simulink model "LgV2"  (Simulink 7.3)
settings: Solver=ode5  StartTime=0.0  StopTime=inf  FixedStep=0.1  RelTol=1e-3
undefined symbols (not defined in the file): eta1_0_real, v1_0_real, velocitySatValues1
libraries: simulink x35, dspmtrx3 x21, simulink_extras x13, dspindex x5, marine_gnc x4, dspinverses x2
(part 2 of 5)

== system LgV2/Control Systems/LgV design 2/Auxilary functions g_q ==
  f_q : Inport
  psi_los^q : Inport  Port=2
  f_q^q : Inport  Port=3
  psi_los^q^2 : Inport  Port=4
  f_q^s : Inport  Port=5
  psi_los^qs : Inport  Port=6
  f_q^t : Inport  Port=7
  g_q eq : Subsystem
  g_q^q eq : Subsystem
  g_q^s eq : Subsystem
  g_q^t eq : Subsystem
  g_q : Outport
  g_q^t : Outport  Port=2
  g_q^q : Outport  Port=3
  g_q^s : Outport  Port=4
  wires:
  g_q eq/1(g_q) -> g_q/1
  psi_los^q/1 -> g_q eq/2(psi_los^q), g_q^q eq/2(psi_los^q), g_q^s eq/2(psi_los^q), g_q^t eq/1(psi_los^q)
  f_q/1 -> g_q eq/1(f_q), g_q^q eq/1(f_q), g_q^s eq/1(f_q)
  f_q^q/1 -> g_q^q eq/3(f_q^q)
  psi_los^q^2/1 -> g_q^q eq/4(psi_los^q^2)
  g_q^q eq/1(g_q^q) -> g_q^q/1
  g_q^s eq/1(g_q^s) -> g_q^s/1
  f_q^s/1 -> g_q^s eq/3(f_q^s)
  psi_los^qs/1 -> g_q^s eq/4(psi_los^qs)
  g_q^t eq/1(g_q^t) -> g_q^t/1
  f_q^t/1 -> g_q^t eq/2(f_q^t)

== system LgV2/Control Systems/LgV design 2/Auxiliary function g_s ==
  psi_los^sq : Inport
  f_s : Inport  Port=2
  psi_los^s : Inport  Port=3
  f_s^q : Inport  Port=4
  f_s^s : Inport  Port=5
  psi_los^s^2 : Inport  Port=6
  f_s^t : Inport  Port=7
  g_s eq : Subsystem
  g_s^q eq : Subsystem
  g_s^s eq : Subsystem
  g_s^t eq : Subsystem
  g_s^q : Outport
  g_s^s : Outport  Port=2
  g_s^t : Outport  Port=3
  g_s : Outport  Port=4
  wires:
  f_s/1 -> g_s eq/1(f_s), g_s^q eq/1(f_s), g_s^s eq/1(f_s)
  psi_los^s/1 -> g_s eq/2(psi_los^s), g_s^q eq/2(psi_los^s), g_s^s eq/2(psi_los^s), g_s^t eq/1(psi_los^s)
  g_s eq/1(g_s) -> g_s/1
  f_s^q/1 -> g_s^q eq/3(f_s^q)
  psi_los^sq/1 -> g_s^q eq/4(psi_los^sq)
  g_s^q eq/1(g_s^q) -> g_s^q/1
  g_s^s eq/1(g_s^s) -> g_s^s/1
  f_s^s/1 -> g_s^s eq/3(f_s^s)
  psi_los^s^2/1 -> g_s^s eq/4(psi_los^s^2)
  g_s^t eq/1(g_a^t) -> g_s^t/1
  f_s^t/1 -> g_s^t eq/2(f_s^t)

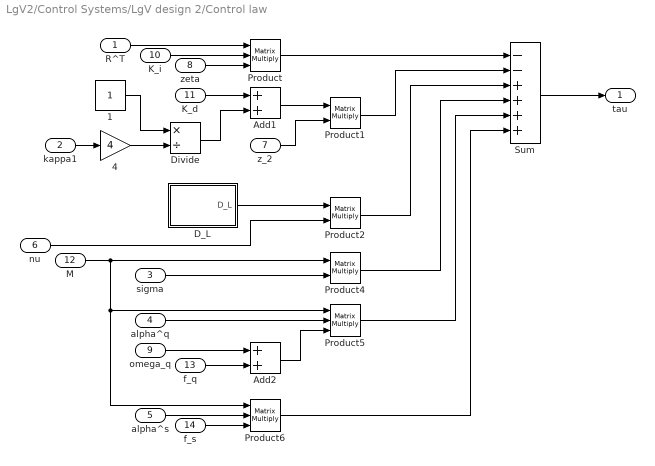
== system LgV2/Control Systems/LgV design 2/Control law ==
  R^T : Inport
  kappa1 : Inport  Port=2
  sigma : Inport  Port=3
  alpha^q : Inport  Port=4
  alpha^s : Inport  Port=5
  nu : Inport  Port=6
  z_2 : Inport  Port=7
  zeta : Inport  Port=8
  omega_q : Inport  Port=9
  K_i : Inport  Port=10
  K_d : Inport  Port=11
  M : Inport  Port=12
  f_q : Inport  Port=13
  f_s : Inport  Port=14
  1 : Constant  OutDataType=fixdt(1, 16)  OutScaling=2^0
  4 : Gain  Gain=4  ParameterDataType=fixdt(1, 16)  ParameterScaling=2^0  OutDataType=fixdt(1, 16)  OutScaling=2^0
  Add1 : Sum  OutDataType=fixdt(1, 16)  OutScaling=2^-10
  Add2 : Sum  OutDataType=fixdt(1, 16)  OutScaling=2^-10
  D_L : Subsystem
  Divide : Product  Inputs=*/  OutDataType=fixdt(1, 16)  OutScaling=2^-10
  Product : Product  Inputs=3  Multiplication=Matrix(*)  OutDataType=fixdt(1, 16)  OutScaling=2^0  RndMeth=Zero
  Product1 : Product  Multiplication=Matrix(*)  OutDataType=fixdt(1, 16)  OutScaling=2^0  RndMeth=Zero
  Product2 : Product  Multiplication=Matrix(*)  OutDataType=fixdt(1, 16)  OutScaling=2^0  RndMeth=Zero
  Product4 : Product  Multiplication=Matrix(*)  OutDataType=fixdt(1, 16)  OutScaling=2^0  RndMeth=Zero
  Product5 : Product  Inputs=3  Multiplication=Matrix(*)  OutDataType=fixdt(1, 16)  OutScaling=2^0  RndMeth=Zero
  Product6 : Product  Inputs=3  Multiplication=Matrix(*)  OutDataType=fixdt(1, 16)  OutScaling=2^0  RndMeth=Zero
  Sum : Sum  Inputs=--++++  OutDataType=fixdt(1, 16)  OutScaling=2^-10
  tau : Outport
  wires:
  Sum/1 -> tau/1
  R^T/1 -> Product/1
  K_i/1 -> Product/2
  zeta/1 -> Product/3
  K_d/1 -> Add1/1
  Divide/1 -> Add1/2
  1/1 -> Divide/1
  kappa1/1 -> 4/1
  4/1 -> Divide/2
  Add1/1 -> Product1/1
  z_2/1 -> Product1/2
  Product1/1 -> Sum/2
  nu/1 -> Product2/2
  D_L/1(D_L) -> Product2/1
  Product2/1 -> Sum/3
  M/1 -> Product4/1, Product5/1, Product6/1
  sigma/1 -> Product4/2
  Product4/1 -> Sum/4
  alpha^q/1 -> Product5/2
  Product5/1 -> Sum/5
  alpha^s/1 -> Product6/2
  f_s/1 -> Product6/3
  Product6/1 -> Sum/6
  omega_q/1 -> Add2/1
  f_q/1 -> Add2/2
  Add2/1 -> Product5/3
  Product/1 -> Sum/1

== system LgV2/Control Systems/LgV design 2/Gamma_q ==
  11 : Inport
  22 : Inport  Port=2
  12 : Constant  Value=0
  21 : Constant  Value=0
  2x2 : Reshape  OutputDimensionality=Customize  OutputDimensions=[2,2]
  Mux : Mux
  Gamma_q : Outport
  wires:
  2x2/1 -> Gamma_q/1
  Mux/1 -> 2x2/1
  11/1 -> Mux/1
  21/1 -> Mux/2
  12/1 -> Mux/3
  22/1 -> Mux/4

== system LgV2/Control Systems/LgV design 2/Integral action state ==
  z_2 : Inport
  R : Inport  Port=2
  Integrator : Integrator  InitialCondition=[0 0 0]'
  Product : Product  Multiplication=Matrix(*)  OutDataType=fixdt(1, 16)  OutScaling=2^0  RndMeth=Zero
  zeta : Outport
  wires:
  R/1 -> Product/1
  z_2/1 -> Product/2
  Integrator/1 -> zeta/1
  Product/1 -> Integrator/1

== system LgV2/Control Systems/LgV design 2/K_d ==
  11 : Inport
  22 : Inport  Port=2
  33 : Inport  Port=3
  {12..13,21,23,31..32} (6 alike) : Constant  Value=0
  3x3 : Reshape  OutputDimensionality=Customize  OutputDimensions=[3,3]
  Mux : Mux  Inputs=9
  K_d : Outport
  wires:
  3x3/1 -> K_d/1
  Mux/1 -> 3x3/1
  11/1 -> Mux/1
  21/1 -> Mux/2
  31/1 -> Mux/3
  12/1 -> Mux/4
  22/1 -> Mux/5
  32/1 -> Mux/6
  13/1 -> Mux/7
  23/1 -> Mux/8
  33/1 -> Mux/9

== system LgV2/Control Systems/LgV design 2/K_i ==
  11 : Inport
  22 : Inport  Port=2
  33 : Inport  Port=3
  {12..13,21,23,31..32} (6 alike) : Constant  Value=0
  3x3 : Reshape  OutputDimensionality=Customize  OutputDimensions=[3,3]
  Mux : Mux  Inputs=9
  K_i : Outport
  wires:
  3x3/1 -> K_i/1
  Mux/1 -> 3x3/1
  11/1 -> Mux/1
  21/1 -> Mux/2
  31/1 -> Mux/3
  12/1 -> Mux/4
  22/1 -> Mux/5
  32/1 -> Mux/6
  13/1 -> Mux/7
  23/1 -> Mux/8
  33/1 -> Mux/9

== system LgV2/Control Systems/LgV design 2/K_p ==
  11 : Inport
  22 : Inport  Port=2
  33 : Inport  Port=3
  {12..13,21,23,31..32} (6 alike) : Constant  Value=0
  Mux : Mux  Inputs=9
  R(psi) : Reshape  OutputDimensionality=Customize  OutputDimensions=[3,3]
  K_p : Outport
  wires:
  R(psi)/1 -> K_p/1
  Mux/1 -> R(psi)/1
  11/1 -> Mux/1
  21/1 -> Mux/2
  31/1 -> Mux/3
  12/1 -> Mux/4
  22/1 -> Mux/5
  32/1 -> Mux/6
  13/1 -> Mux/7
  23/1 -> Mux/8
  33/1 -> Mux/9

== system LgV2/Control Systems/LgV design 2/M ==
  3x3 : Reshape  OutputDimensionality=Customize  OutputDimensions=[3,3]
  I_z : Constant  Value=1.760
  M_{11,22..23,32..33} (5 alike) : Sum  Inputs=+-
  M_{12..13,21,31} (4 alike) : Constant  Value=0
  Mux : Mux  Inputs=9
  N_rdot : Constant  Value=-1.0
  N_vdot : Constant  Value=-0.0
  X_udot : Constant  Value=-2.0
  Y_rdot : Constant  Value=0.0
  Y_vdot : Constant  Value=-10.0
  m : Constant  Value=17.6
  m x_g : Product  RndMeth=Zero
  x_g : Constant  Value=0.03
  M : Outport
  wires:
  3x3/1 -> M/1
  Mux/1 -> 3x3/1
  M_33/1 -> Mux/9
  M_23/1 -> Mux/8
  M_13/1 -> Mux/7
  M_32/1 -> Mux/6
  M_22/1 -> Mux/5
  M_12/1 -> Mux/4
  M_31/1 -> Mux/3
  M_21/1 -> Mux/2
  M_11/1 -> Mux/1
  N_rdot/1 -> M_33/2
  I_z/1 -> M_33/1
  Y_rdot/1 -> M_23/2
  N_vdot/1 -> M_32/2
  m x_g/1 -> M_23/1, M_32/1
  x_g/1 -> m x_g/2
  Y_vdot/1 -> M_22/2
  X_udot/1 -> M_11/2
  m/1 -> m x_g/1, M_22/1, M_11/1

== system LgV2/Control Systems/LgV design 2/R(psi) ==
  psi : Inport
  -1 : Gain  Gain=-1  ParameterDataType=fixdt(1, 16)  ParameterScaling=2^0  OutDataType=fixdt(1, 16)  OutScaling=2^0
  Mux : Mux  Inputs=9
  R(psi) : Reshape  OutputDimensionality=Customize  OutputDimensions=[3,3]
  R11 : Trigonometry  Operator=cos
  R12 : Trigonometry
  R{13,23,31..32} (4 alike) : Constant  Value=0
  R21 : Trigonometry
  R22 : Trigonometry  Operator=cos
  R33 : Constant
  R : Outport
  wires:
  R(psi)/1 -> R/1
  Mux/1 -> R(psi)/1
  psi/1 -> R11/1, R21/1, R12/1, R22/1
  R11/1 -> Mux/1
  R21/1 -> Mux/2
  R31/1 -> Mux/3
  R12/1 -> -1/1
  R22/1 -> Mux/5
  R32/1 -> Mux/6
  R13/1 -> Mux/7
  R33/1 -> Mux/9
  R23/1 -> Mux/8
  -1/1 -> Mux/4

== system LgV2/Control Systems/LgV design 2/S(r) ==
  r : Inport
  Mux : Mux  Inputs=9
  R31 : Constant  Value=0
  S(r) : Reshape  OutputDimensionality=Customize  OutputDimensions=[3,3]
  S{11,13,22..23,32} (5 alike) : Constant  Value=0
  S12 : Gain  ParameterDataType=fixdt(1, 16)  ParameterScaling=2^0  OutDataType=fixdt(1, 16)  OutScaling=2^0
  S33 : Constant
  S : Outport
  wires:
  S(r)/1 -> S/1
  Mux/1 -> S(r)/1
  R31/1 -> Mux/3
  S12/1 -> Mux/4
  S22/1 -> Mux/5
  S32/1 -> Mux/6
  S13/1 -> Mux/7
  S33/1 -> Mux/9
  S23/1 -> Mux/8
  r/1 -> Mux/2, S12/1
  S11/1 -> Mux/1

== system LgV2/Control Systems/LgV design 2/Thruster allocation ==
  tau : Inport
  f_act to u_act : Subsystem
  tau to f_act : Subsystem
  u_act : Outport
  wires:
  tau/1 -> tau to f_act/1(tau)
  tau to f_act/1(f_act) -> f_act to u_act/1(f_act)
  f_act to u_act/1(u_act) -> u_act/1

== system LgV2/Control Systems/LgV design 2/Update laws ==
  V_1^q : Inport
  Gamma_q : Inport  Port=2
  lambda : Inport  Port=3
  f_q : Inport  Port=4
  f_s : Inport  Port=5
  Add : Sum  OutDataType=fixdt(1, 16)  OutScaling=2^-10
  Add1 : Sum  OutDataType=fixdt(1, 16)  OutScaling=2^-10
  Gain : Gain  Gain=-1  ParameterDataType=fixdt(1, 16)  ParameterScaling=2^0  OutDataType=fixdt(1, 16)  OutScaling=2^0
  Integrator : Integrator  ExternalReset=level  InitialConditionSource=external
  Integrator1 : Integrator  ExternalReset=level  InitialConditionSource=external  InitialCondition=250
  Integrator2 : Integrator  ExternalReset=level
  Product : Product  Multiplication=Matrix(*)  OutDataType=fixdt(1, 16)  OutScaling=2^0  RndMeth=Zero
  Product1 : Product  OutDataType=fixdt(1, 16)  OutScaling=2^0  RndMeth=Zero
  Reset omega_q : Constant  Value=0
  Reset q : Constant  Value=0
  Reset s : Constant  Value=0
  Transpose : dspmtrx3/Transpose  SystemSampleTime=-1  Hermitian=off  overflowFlag=off
  q_0 : Subsystem
  s_0 : Constant  Value=0
  omega_q : Outport
  q : Outport  Port=2  PortDimensions=2
  s : Outport  Port=3  PortDimensions=1
  wires:
  f_q/1 -> Add/2
  Add/1 -> Integrator/1
  Product/1 -> Add1/2
  V_1^q/1 -> Transpose/1
  Gamma_q/1 -> Product/1
  lambda/1 -> Product1/1
  Add1/1 -> Product1/2
  Product1/1 -> Gain/1
  Gain/1 -> Integrator2/1
  f_s/1 -> Integrator1/1
  Transpose/1 -> Product/2
  Integrator/1 -> q/1
  Integrator1/1 -> s/1
  Integrator2/1 -> omega_q/1, Add/1, Add1/1
  Reset s/1 -> Integrator1/2
  s_0/1 -> Integrator1/3
  Reset q/1 -> Integrator/2
  q_0/1(q_0) -> Integrator/3
  Reset omega_q/1 -> Integrator2/2

== system LgV2/Control Systems/LgV design 2/V_1^q ==
  chi^q : Inport
  z_1 : Inport  Port=2
  R^T : Inport  Port=3
  Gain : Gain  Gain=-1  ParameterDataType=fixdt(1, 16)  ParameterScaling=2^0  OutDataType=fixdt(1, 16)  OutScaling=2^0
  Product : Product  Inputs=3  Multiplication=Matrix(*)  OutDataType=fixdt(1, 16)  OutScaling=2^0  RndMeth=Zero
  Transpose : dspmtrx3/Transpose  SystemSampleTime=-1  Hermitian=off  overflowFlag=off
  V_1^q : Outport
  wires:
  Product/1 -> Gain/1
  R^T/1 -> Product/2
  z_1/1 -> Transpose/1
  Transpose/1 -> Product/1
  chi^q/1 -> Product/3
  Gain/1 -> V_1^q/1

== system LgV2/Control Systems/LgV design 2/Virtual control ==
  g_q : Inport
  g_s : Inport  Port=2
  K_p : Inport  Port=3
  kappa_1 : Inport  Port=4
  R^T : Inport  Port=5
  z_1 : Inport  Port=6
  Add : Sum  OutDataType=fixdt(1, 16)  OutScaling=2^-10
  I : dspmtrx3/Constant Diagonal Matrix  SystemSampleTime=-1  q=[1 1 1 ]  frame=off  dataType=Inherit from 'Constant(s) along diagonal'  isSigned=on  wordLen=16  udDataType=sfix(16)  fracBitsMode=Best precision  numFracBits=15
  Product : Product  OutDataType=fixdt(1, 16)  OutScaling=2^0  RndMeth=Zero
  Product1 : Product  Multiplication=Matrix(*)  OutDataType=fixdt(1, 16)  OutScaling=2^0  RndMeth=Zero
  Product2 : Product  Multiplication=Matrix(*)  OutDataType=fixdt(1, 16)  OutScaling=2^0  RndMeth=Zero
  Subtract : Sum  Inputs=+-  OutDataType=fixdt(1, 16)  OutScaling=2^-10
  Sum : Sum  Inputs=-+  OutDataType=fixdt(1, 16)  OutScaling=2^-10
  alpha : Outport
  wires:
  Sum/1 -> alpha/1
  K_p/1 -> Subtract/1
  kappa_1/1 -> Product/1
  I/1 -> Product/2
  Product/1 -> Subtract/2
  Subtract/1 -> Product1/1
  z_1/1 -> Product1/2
  Product1/1 -> Sum/1
  R^T/1 -> Product2/1
  g_q/1 -> Add/1
  g_s/1 -> Add/2
  Add/1 -> Product2/2
  Product2/1 -> Sum/2

== system LgV2/Control Systems/LgV design 2/alpha^q ==
  kappa1 : Inport
  R^T : Inport  Port=2
  K_p : Inport  Port=3
  g_q^q : Inport  Port=4
  g_s^q : Inport  Port=5
  chi^q : Inport  Port=6
  Add : Sum  OutDataType=fixdt(1, 16)  OutScaling=2^-10
  Add2 : Sum  OutDataType=fixdt(1, 16)  OutScaling=2^-10
  Add3 : Sum  OutDataType=fixdt(1, 16)  OutScaling=2^-10
  I : dspmtrx3/Constant Diagonal Matrix  SystemSampleTime=-1  q=[1 1 1 ]  frame=off  dataType=Inherit from 'Constant(s) along diagonal'  isSigned=on  wordLen=16  udDataType=sfix(16)  fracBitsMode=Best precision  numFracBits=15
  Product1 : Product  OutDataType=fixdt(1, 16)  OutScaling=2^0  RndMeth=Zero
  Product3 : Product  Inputs=3  Multiplication=Matrix(*)  OutDataType=fixdt(1, 16)  OutScaling=2^0  RndMeth=Zero
  Product4 : Product  Multiplication=Matrix(*)  OutDataType=fixdt(1, 16)  OutScaling=2^0  RndMeth=Zero
  alpha^q : Outport
  wires:
  Add3/1 -> alpha^q/1
  K_p/1 -> Add/1
  Product1/1 -> Add/2
  kappa1/1 -> Product1/1
  I/1 -> Product1/2
  Add/1 -> Product3/1
  g_q^q/1 -> Add2/1
  g_s^q/1 -> Add2/2
  Add2/1 -> Product4/2
  R^T/1 -> Product3/2, Product4/1
  chi^q/1 -> Product3/3
  Product3/1 -> Add3/1
  Product4/1 -> Add3/2

== system LgV2/Control Systems/LgV design 2/alpha^s ==
  kappa1 : Inport
  R^T : Inport  Port=2
  K_p : Inport  Port=3
  g_q^s : Inport  Port=4
  g_s^s : Inport  Port=5
  chi^s : Inport  Port=6
  Add1 : Sum  OutDataType=fixdt(1, 16)  OutScaling=2^-10
  Add2 : Sum  OutDataType=fixdt(1, 16)  OutScaling=2^-10
  Add3 : Sum  OutDataType=fixdt(1, 16)  OutScaling=2^-10
  I : dspmtrx3/Constant Diagonal Matrix  SystemSampleTime=-1  q=[1 1 1 ]  frame=off  dataType=Inherit from 'Constant(s) along diagonal'  isSigned=on  wordLen=16  udDataType=sfix(16)  fracBitsMode=Best precision  numFracBits=15
  Product1 : Product  OutDataType=fixdt(1, 16)  OutScaling=2^0  RndMeth=Zero
  Product3 : Product  Inputs=3  Multiplication=Matrix(*)  OutDataType=fixdt(1, 16)  OutScaling=2^0  RndMeth=Zero
  Product4 : Product  Multiplication=Matrix(*)  OutDataType=fixdt(1, 16)  OutScaling=2^0  RndMeth=Zero
  alpha^s : Outport
  wires:
  Add3/1 -> alpha^s/1
  K_p/1 -> Add1/1
  Product1/1 -> Add1/2
  kappa1/1 -> Product1/1
  I/1 -> Product1/2
  Add1/1 -> Product3/1
  g_q^s/1 -> Add2/1
  g_s^s/1 -> Add2/2
  Add2/1 -> Product4/2
  R^T/1 -> Product3/2, Product4/1
  chi^s/1 -> Product3/3
  Product3/1 -> Add3/1
  Product4/1 -> Add3/2

== system LgV2/Control Systems/LgV design 2/sigma eq ==
  kappa1 : Inport
  R^T : Inport  Port=2
  K_p : Inport  Port=3
  S^T : Inport  Port=4
  g_q : Inport  Port=5
  nu : Inport  Port=6
  g_q^t : Inport  Port=7
  g_s : Inport  Port=8
  g_s^t : Inport  Port=9
  z_1 : Inport  Port=10
  Add{,1..3} (4 alike) : Sum  OutDataType=fixdt(1, 16)  OutScaling=2^-10
  I : dspmtrx3/Constant Diagonal Matrix  SystemSampleTime=-1  q=[1 1 1 ]  frame=off  dataType=Inherit from 'Constant(s) along diagonal'  isSigned=on  wordLen=16  udDataType=sfix(16)  fracBitsMode=Best precision  numFracBits=15
  Product : Product  Multiplication=Matrix(*)  OutDataType=fixdt(1, 16)  OutScaling=2^0  RndMeth=Zero
  Product1 : Product  OutDataType=fixdt(1, 16)  OutScaling=2^0  RndMeth=Zero
  Product2 : Product  Multiplication=Matrix(*)  OutDataType=fixdt(1, 16)  OutScaling=2^0  RndMeth=Zero
  Product3 : Product  Inputs=3  Multiplication=Matrix(*)  OutDataType=fixdt(1, 16)  OutScaling=2^0  RndMeth=Zero
  Product4 : Product  Multiplication=Matrix(*)  OutDataType=fixdt(1, 16)  OutScaling=2^0  RndMeth=Zero
  Sum : Sum  Inputs=-++  OutDataType=fixdt(1, 16)  OutScaling=2^-10
  sigma : Outport
  wires:
  Sum/1 -> sigma/1
  K_p/1 -> Add3/1
  Product1/1 -> Add3/2
  kappa1/1 -> Product1/1
  I/1 -> Product1/2
  S^T/1 -> Product/1, Product3/1
  z_1/1 -> Product/2
  Product/1 -> Add/1
  nu/1 -> Add/2
  Add3/1 -> Product2/1
  Add/1 -> Product2/2
  Product2/1 -> Sum/1
  g_q/1 -> Add1/1
  g_s/1 -> Add1/2
  g_q^t/1 -> Add2/1
  g_s^t/1 -> Add2/2
  R^T/1 -> Product3/2, Product4/1
  Add1/1 -> Product3/3
  Add2/1 -> Product4/2
  Product3/1 -> Sum/2
  Product4/1 -> Sum/3

== system LgV2/Control Systems/LgV design 2/z_1 eq ==
  eta : Inport
  chi : Inport  Port=2
  R^T : Inport  Port=3
  Product : Product  Multiplication=Matrix(*)  OutDataType=fixdt(1, 16)  OutScaling=2^0  RndMeth=Zero
  Subtract : Sum  Inputs=+-  OutDataType=fixdt(1, 16)  OutScaling=2^-10
  heading to pipi : Subsystem
  heading to pipi1 : Subsystem
  z_1 : Outport
  wires:
  R^T/1 -> Product/1
  eta/1 -> heading to pipi/1(In1)
  chi/1 -> Subtract/2
  Subtract/1 -> heading to pipi1/1(In1)
  Product/1 -> z_1/1
  heading to pipi/1(Out1) -> Subtract/1
  heading to pipi1/1(Out1) -> Product/2

== system LgV2/Control Systems/LgV design 2/z_2 eq ==
  nu : Inport
  alpha : Inport  Port=2
  Subtract : Sum  Inputs=+-  OutDataType=fixdt(1, 16)  OutScaling=2^-10
  z_2 : Outport
  wires:
  nu/1 -> Subtract/1
  alpha/1 -> Subtract/2
  Subtract/1 -> z_2/1

== system LgV2/Control Systems/PS3 u input control/Subsystem ==
  u_act : Inport  OutDataType=fixdt(1, 16)  OutScaling=2^0
  Bus Selector : BusSelector  OutputSignals=u_1,u_2,u_3,u_4,u_5
  Mux : Mux  Inputs=5
  f_act to tau : Subsystem
  u_act to f_act : Subsystem
  tau : Outport
  wires:
  u_act/1 -> Bus Selector/1
  f_act to tau/1(tau) -> tau/1
  u_act to f_act/1(f_act) -> f_act to tau/1(f_act)
  Mux/1 -> u_act to f_act/1(u_act)
  Bus Selector/1 -> Mux/1  "<u_1>"
  Bus Selector/2 -> Mux/2  "<u_2>"
  Bus Selector/3 -> Mux/3  "<u_3>"
  Bus Selector/4 -> Mux/4  "<u_4>"
  Bus Selector/5 -> Mux/5  "<u_5>"

== system LgV2/Guidance Systems/Path-following/Heading ==
  p_d^s : Inport
  p_d^s^2 : Inport  Port=2
  p_d^s^3 : Inport  Port=3
  Demux : Demux  Outputs=2
  Demux1 : Demux  Outputs=2
  Demux2 : Demux  Outputs=2
  psi_d eq : Subsystem
  psi_d^s eq : Subsystem
  psi_d^s^2 eq : Subsystem
  psi_d : Outport
  psi_d^s : Outport  Port=2
  psi_d^s^2 : Outport  Port=3
  wires:
  psi_d eq/1(psi_d) -> psi_d/1
  Demux/1 -> psi_d eq/1(x_d^s), psi_d^s eq/1(x_d^s), psi_d^s^2 eq/3(x_d^s)
  Demux/2 -> psi_d eq/2(y_d^s), psi_d^s eq/2(y_d^s), psi_d^s^2 eq/4(y_d^s)
  p_d^s/1 -> Demux/1
  p_d^s^2/1 -> Demux1/1
  Demux1/1 -> psi_d^s eq/3(x_d^s^2), psi_d^s^2 eq/5(x_d^s^2)
  Demux1/2 -> psi_d^s eq/4(y_d^s^2), psi_d^s^2 eq/6(y_d^s^2)
  psi_d^s eq/1(psi_d^s) -> psi_d^s/1
  p_d^s^3/1 -> Demux2/1
  psi_d^s^2 eq/1(psi_d^s^2) -> psi_d^s^2/1
  Demux2/1 -> psi_d^s^2 eq/7(x_d^s^3)
  Demux2/2 -> psi_d^s^2 eq/8(y_d^s^3)
  psi_d^s eq/2(num) -> psi_d^s^2 eq/1(num)
  psi_d^s eq/3(den) -> psi_d^s^2 eq/2(den)

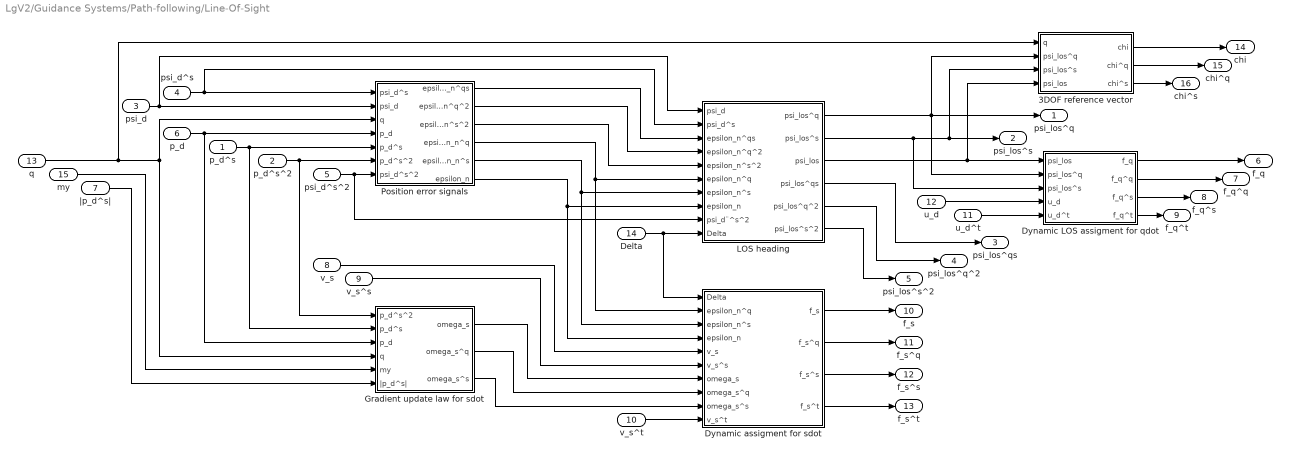
== system LgV2/Guidance Systems/Path-following/Line-Of-Sight ==
  p_d^s : Inport
  p_d^s^2 : Inport  Port=2
  psi_d : Inport  Port=3
  psi_d^s : Inport  Port=4
  psi_d^s^2 : Inport  Port=5
  p_d : Inport  Port=6
  |p_d^s| : Inport  Port=7
  v_s : Inport  Port=8
  v_s^s : Inport  Port=9
  v_s^t : Inport  Port=10
  u_d^t : Inport  Port=11
  u_d : Inport  Port=12
  q : Inport  Port=13
  Delta : Inport  Port=14
  my : Inport  Port=15
  3DOF reference vector : Subsystem
  Dynamic LOS assigment for qdot : Subsystem
  Dynamic assigment for sdot : Subsystem
  Gradient update law for sdot : Subsystem
  LOS heading : Subsystem
  Position error signals : Subsystem
  psi_los^q : Outport
  psi_los^s : Outport  Port=2
  psi_los^qs : Outport  Port=3
  psi_los^q^2 : Outport  Port=4
  psi_los^s^2 : Outport  Port=5
  f_q : Outport  Port=6
  "f_q^q " : Outport  Port=7
  f_q^s : Outport  Port=8
  f_q^t : Outport  Port=9
  f_s : Outport  Port=10
  f_s^q : Outport  Port=11
  f_s^s : Outport  Port=12
  f_s^t : Outport  Port=13
  chi : Outport  Port=14
  chi^q : Outport  Port=15
  chi^s : Outport  Port=16
  wires:
  Dynamic assigment for sdot/1(f_s) -> f_s/1
  Delta/1 -> Dynamic assigment for sdot/1(Delta), LOS heading/10(Delta)
  psi_d/1 -> Position error signals/2(psi_d), LOS heading/1(psi_d)
  v_s/1 -> Dynamic assigment for sdot/5(v_s)
  Gradient update law for sdot/1(omega_s) -> Dynamic assigment for sdot/7(omega_s)
  p_d^s/1 -> Gradient update law for sdot/2(p_d^s), Position error signals/5(p_d^s)
  my/1 -> Gradient update law for sdot/5(my)
  |p_d^s|/1 -> Gradient update law for sdot/6(|p_d^s|)
  u_d/1 -> Dynamic LOS assigment for qdot/4(u_d)
  LOS heading/3(psi_los) -> Dynamic LOS assigment for qdot/1(psi_los), 3DOF reference vector/4(psi_los)
  p_d/1 -> Position error signals/4(p_d), Gradient update law for sdot/3(p_d)
  q/1 -> Position error signals/3(q), Gradient update law for sdot/4(q), 3DOF reference vector/1(q)
  Position error signals/6(epsilon_n) -> Dynamic assigment for sdot/4(epsilon_n), LOS heading/8(epsilon_n)
  Position error signals/5(epsilon_n^s) -> LOS heading/7(epsilon_n^s), Dynamic assigment for sdot/3(epsilon_n^s)
  Position error signals/1(epsilon_n^qs) -> LOS heading/3(epsilon_n^qs)
  Position error signals/2(epsilon_n^q^2) -> LOS heading/4(epsilon_n^q^2)
  Position error signals/3(epsilon_n^s^2) -> LOS heading/5(epsilon_n^s^2)
  psi_d^s/1 -> Position error signals/1(psi_d^s), LOS heading/2(psi_d^s)
  Position error signals/4(epsilon_n^q) -> LOS heading/6(epsilon_n^q), Dynamic assigment for sdot/2(epsilon_n^q)
  LOS heading/1(psi_los^q) -> 3DOF reference vector/2(psi_los^q), Dynamic LOS assigment for qdot/2(psi_los^q), psi_los^q/1
  LOS heading/2(psi_los^s) -> Dynamic LOS assigment for qdot/3(psi_los^s), 3DOF reference vector/3(psi_los^s), psi_los^s/1
  3DOF reference vector/1(chi) -> chi/1
  3DOF reference vector/2(chi^q) -> chi^q/1
  3DOF reference vector/3(chi^s) -> chi^s/1
  Dynamic LOS assigment for qdot/2("f_q^q ") -> "f_q^q "/1
  Dynamic LOS assigment for qdot/3(f_q^s) -> f_q^s/1
  Dynamic LOS assigment for qdot/4(f_q^t) -> f_q^t/1
  p_d^s^2/1 -> Position error signals/6(p_d^s^2), Gradient update law for sdot/1(p_d^s^2)
  Dynamic LOS assigment for qdot/1(f_q) -> f_q/1
  v_s^s/1 -> Dynamic assigment for sdot/6(v_s^s)
  Gradient update law for sdot/2(omega_s^q) -> Dynamic assigment for sdot/8(omega_s^q)
  Gradient update law for sdot/3(omega_s^s) -> Dynamic assigment for sdot/9(omega_s^s)
  psi_d^s^2/1 -> Position error signals/7(psi_d^s^2), LOS heading/9(psi_d¨^s^2)
  Dynamic assigment for sdot/4(f_s^t) -> f_s^t/1
  Dynamic assigment for sdot/3(f_s^s) -> f_s^s/1
  Dynamic assigment for sdot/2(f_s^q) -> f_s^q/1
  LOS heading/4(psi_los^qs) -> psi_los^qs/1
  LOS heading/5(psi_los^q^2) -> psi_los^q^2/1
  LOS heading/6(psi_los^s^2) -> psi_los^s^2/1
  u_d^t/1 -> Dynamic LOS assigment for qdot/5(u_d^t)
  v_s^t/1 -> Dynamic assigment for sdot/10(v_s^t)

== system LgV2/Guidance Systems/Path-following/Path ==
  note: Path Selector == 1: Straight path
      | Path Selector == 0: Ellipse path
  s : Inport
  x_1 : Inport  Port=2
  y_1 : Inport  Port=3
  x_2 : Inport  Port=4
  y_2 : Inport  Port=5
  origo_x : Inport  Port=6
  origo_y : Inport  Port=7
  r_x : Inport  Port=8
  r_y : Inport  Port=9
  k : Inport  Port=10
  Ellipse path : Subsystem
  Path Selector : Constant  Value=0
  Path Switch workaround : Subsystem
  Straight path : Subsystem
  saturation : Subsystem
  p_d^s : Outport
  p_d^s^2 : Outport  Port=2
  p_d^s^3 : Outport  Port=3
  p_d : Outport  Port=4
  |p_d^s| : Outport  Port=5
  path : Outport  Port=6
  wires:
  s/1 -> Straight path/1(s), Ellipse path/1(s)
  x_2/1 -> Straight path/4(x_2)
  y_2/1 -> Straight path/5(y_2)
  x_1/1 -> Straight path/2(x_1)
  y_1/1 -> Straight path/3(y1)
  r_x/1 -> Ellipse path/4(r_x)
  r_y/1 -> Ellipse path/5(r_y)
  origo_x/1 -> Ellipse path/2(origo_x)
  origo_y/1 -> Ellipse path/3(origo_y)
  Path Selector/1 -> Path Switch workaround/1(Path Selector), path/1  "chosen path"
  Straight path/1(p_d) -> Path Switch workaround/2(p_d Straight path)  "p_d"
  Straight path/2(p_d^s) -> Path Switch workaround/3(p_d^s Straight path)  "p_d^s"
  Straight path/3(p_d^s^2) -> Path Switch workaround/4(p_d^s^3 Straight path)  "p_d^s^2"
  Straight path/4(p_d^s^3) -> Path Switch workaround/5(p_d^s^2 Straight path)  "p_d^s^3"
  Straight path/5(|p_d^s|) -> Path Switch workaround/6(|p_d^s| Straight path)  "|p_d^s|"
  Ellipse path/1(p_d) -> Path Switch workaround/7(p_d Ellipse path)
  Ellipse path/2(p_d^s) -> Path Switch workaround/8(p_d^s Ellipse path)
  Ellipse path/3(p_d^s^2) -> Path Switch workaround/9(p_d^s^3 Ellipse path)
  Ellipse path/4(p_d^s^3) -> Path Switch workaround/10(p_d^s^2 Ellipse path)
  Ellipse path/5(|p_d^s|) -> Path Switch workaround/11(|p_d^s| Ellipse path)
  k/1 -> Ellipse path/6(k)
  saturation/1(sat_p_d) -> p_d/1
  Path Switch workaround/1(p_d) -> saturation/1(p_d)
  Path Switch workaround/2(p_d^s) -> p_d^s/1
  Path Switch workaround/3(p_d^s^2) -> p_d^s^2/1
  Path Switch workaround/4(p_d^s^3) -> p_d^s^3/1
  Path Switch workaround/5(|p_d^s|) -> |p_d^s|/1

== system LgV2/Guidance Systems/Path-following/Speed assigment ==
  |p_d^s| : Inport
  p_d^s : Inport  Port=2
  p_d^s^2 : Inport  Port=3
  u_d : Inport  Port=4
  Derivative : Derivative
  v_s eq : Subsystem
  v_s^s eq : Subsystem
  v_s^t eq : Subsystem
  v_s : Outport
  v_s^s : Outport  Port=2
  v_s^t : Outport  Port=3
  u_d^t : Outport  Port=4
  wires:
  v_s eq/1(v_s) -> v_s/1
  |p_d^s|/1 -> v_s eq/1(|p_d^s|), v_s^s eq/1(|p_d^s|), v_s^t eq/1(|p_d^s|)
  u_d/1 -> v_s eq/2(u_d), v_s^s eq/2(u_d), Derivative/1
  v_s^s eq/1(v_s^s) -> v_s^s/1
  p_d^s/1 -> v_s^s eq/3(p_d^s)
  p_d^s^2/1 -> v_s^s eq/4(p_d^s^2)
  v_s^t eq/1(v_s^t) -> v_s^t/1
  Derivative/1 -> v_s^t eq/2(u_d^t), u_d^t/1

== system LgV2/Plants/CSE1/Bow Thruster ==
  Bow Thruster Direction u_5 : Inport
  Bow Thruster Power : Inport  Port=2
  Add : Sum  Inputs=+++
  BT_D_Gain1 : Gain  Gain=0.02
  BT_D_Gain2 : Gain  Gain=0.02
  BT_L_Gain1 : Gain  Gain=0.02
  BT_L_Gain2 : Gain  Gain=-0.02
  BT_Power_Offset1 : Constant  Value=0.05
  BT_Power_Offset2 : Constant  Value=0.05
  BT_Power_Offset3 : Constant  Value=0.05
  Constant : Constant  Value=0  OutDataType=fixdt(1, 16)  OutScaling=2^0
  Constant1 : Constant  Value=0  OutDataType=fixdt(1, 16)  OutScaling=2^0
  Neg : Gain  Gain=-1  ParameterDataType=fixdt(1, 16)  ParameterScaling=2^0  OutDataType=fixdt(1, 16)  OutScaling=2^0
  SIT PWM0 BT : S-Function  Priority=1  FunctionName=NI_SIT_IO  Parameters=width dtype portnum stime stype btype  EnableBusSupport=off  mask(SIT Outport){portnum=1, width=-1, stime=-1, dtype=auto, stype=auto, btype=0}
      mask prompts: portnum "Port number:"; width "Port dimensions (-1 for dynamically sized):"; stime "Sample time (-1 for inherited):"; dtype "Data type:"; stype "Signal type:"; btype "Block type:"
      mask help: Use this outport on any level of nested subsystems to allow the LabVIEW Simulation Interface Toolkit to map hardware to it.
      mask init:
      | NI_SIT_IO_init;
      settings: CopyFcn=NI_SIT_IO_callbacks(1);  DeleteFcn=NI_SIT_IO_callbacks(2);
      mask StyleString: edit,edit,edit,popup(auto|double|single|int8|uint8|int16|uint16|int32|uint32|boolean),popup(auto|real|complex),edit
      mask CallbackString: NI_SIT_IO_callbacks(3);|||NI_SIT_IO_callbacks(4);||
      mask TabNameString: Parameters,Parameters,Parameters,Parameters,Parameters,Parameters
      mask Display:
      | patch([-x x], [-y y], [.90980 .81960 .32156]);
      | plot([0 -x x 0], [rad -y y rad]);
      | fprintf('SIT%d', portnum);
  Saturation Dynamic : simulink/Discontinuities/Saturation Dynamic  SystemSampleTime=-1  OutMin=[]  OutMax=[]  OutDataTypeStr=Inherit: Same as second input  OutDataType=fixdt(1, 16)  OutScaling=2^-10  DoSatur=off
  Saturation Dynamic1 : simulink/Discontinuities/Saturation Dynamic  SystemSampleTime=-1  OutMin=[]  OutMax=[]  OutDataTypeStr=Inherit: Same as second input  OutDataType=fixdt(1, 16)  OutScaling=2^-10  DoSatur=off
  Saturation Dynamic2 : simulink/Discontinuities/Saturation Dynamic  SystemSampleTime=-1  OutMin=[]  OutMax=[]  OutDataTypeStr=Inherit: Same as second input  OutDataType=fixdt(1, 16)  OutScaling=2^-10  DoSatur=off
  Sum1 : Sum  Inputs=|++
  Sum2 : Sum  Inputs=|++
  Terminator : Terminator
  Terminator1 : Terminator
  wires:
  Bow Thruster Direction u_5/1 -> BT_D_Gain1/1, Saturation Dynamic1/2, BT_D_Gain2/1, Saturation Dynamic2/2
  BT_D_Gain1/1 -> Add/1
  BT_D_Gain2/1 -> Add/3
  BT_Power_Offset1/1 -> Add/2
  Add/1 -> Saturation Dynamic/2
  Bow Thruster Power/1 -> BT_L_Gain2/1, Saturation Dynamic2/1, BT_L_Gain1/1, Neg/1
  Sum1/1 -> Saturation Dynamic/1
  BT_L_Gain1/1 -> Sum1/1
  BT_L_Gain2/1 -> Sum2/1
  Sum2/1 -> Saturation Dynamic/3
  BT_Power_Offset2/1 -> Sum1/2
  BT_Power_Offset3/1 -> Sum2/2
  Saturation Dynamic/1 -> SIT PWM0 BT/1
  Saturation Dynamic2/1 -> Terminator1/1
  Saturation Dynamic1/1 -> Terminator/1
  Constant/1 -> Saturation Dynamic1/1
  Constant1/1 -> Saturation Dynamic2/3
  Neg/1 -> Saturation Dynamic1/3

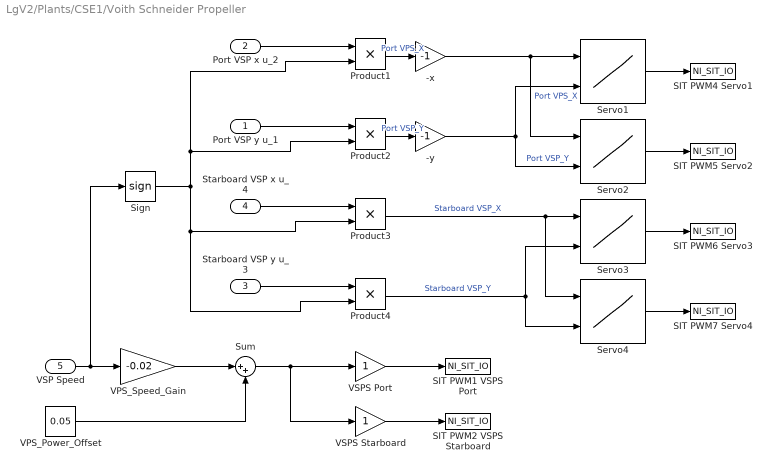
== system LgV2/Plants/CSE1/Voith Schneider Propeller  ==
  Port VSP y u_1 : Inport
  Port VSP x u_2 : Inport  Port=2
  Starboard VSP y u_3 : Inport  Port=3
  Starboard VSP x u_4 : Inport  Port=4
  VSP Speed : Inport  Port=5
  -x : Gain  Gain=-1
  -y : Gain  Gain=-1
  Product{1..4} (4 alike) : Product  RndMeth=Zero
  SIT PWM1 VSPS Port : S-Function  Priority=5  FunctionName=NI_SIT_IO  Parameters=width dtype portnum stime stype btype  EnableBusSupport=off  mask(SIT Outport){portnum=5, width=-1, stime=-1, dtype=auto, stype=auto, btype=0}
      mask prompts: portnum "Port number:"; width "Port dimensions (-1 for dynamically sized):"; stime "Sample time (-1 for inherited):"; dtype "Data type:"; stype "Signal type:"; btype "Block type:"
      mask help: Use this outport on any level of nested subsystems to allow the LabVIEW Simulation Interface Toolkit to map hardware to it.
      mask init:
      | NI_SIT_IO_init;
      settings: CopyFcn=NI_SIT_IO_callbacks(1);  DeleteFcn=NI_SIT_IO_callbacks(2);
      mask StyleString: edit,edit,edit,popup(auto|double|single|int8|uint8|int16|uint16|int32|uint32|boolean),popup(auto|real|complex),edit
      mask CallbackString: NI_SIT_IO_callbacks(3);|||NI_SIT_IO_callbacks(4);||
      mask TabNameString: Parameters,Parameters,Parameters,Parameters,Parameters,Parameters
      mask Display:
      | patch([-x x], [-y y], [.90980 .81960 .32156]);
      | plot([0 -x x 0], [rad -y y rad]);
      | fprintf('SIT%d', portnum);
  SIT PWM2 VSPS Starboard : S-Function  Priority=6  FunctionName=NI_SIT_IO  Parameters=width dtype portnum stime stype btype  EnableBusSupport=off  mask(SIT Outport){portnum=6, width=-1, stime=-1, dtype=auto, stype=auto, btype=0}
      mask prompts: portnum "Port number:"; width "Port dimensions (-1 for dynamically sized):"; stime "Sample time (-1 for inherited):"; dtype "Data type:"; stype "Signal type:"; btype "Block type:"
      mask help: Use this outport on any level of nested subsystems to allow the LabVIEW Simulation Interface Toolkit to map hardware to it.
      mask init:
      | NI_SIT_IO_init;
      settings: CopyFcn=NI_SIT_IO_callbacks(1);  DeleteFcn=NI_SIT_IO_callbacks(2);
      mask StyleString: edit,edit,edit,popup(auto|double|single|int8|uint8|int16|uint16|int32|uint32|boolean),popup(auto|real|complex),edit
      mask CallbackString: NI_SIT_IO_callbacks(3);|||NI_SIT_IO_callbacks(4);||
      mask TabNameString: Parameters,Parameters,Parameters,Parameters,Parameters,Parameters
      mask Display:
      | patch([-x x], [-y y], [.90980 .81960 .32156]);
      | plot([0 -x x 0], [rad -y y rad]);
      | fprintf('SIT%d', portnum);
  SIT PWM4 Servo1 : S-Function  Priority=1  FunctionName=NI_SIT_IO  Parameters=width dtype portnum stime stype btype  EnableBusSupport=off  mask(SIT Outport){portnum=1, width=-1, stime=-1, dtype=auto, stype=auto, btype=0}
      mask prompts: portnum "Port number:"; width "Port dimensions (-1 for dynamically sized):"; stime "Sample time (-1 for inherited):"; dtype "Data type:"; stype "Signal type:"; btype "Block type:"
      mask help: Use this outport on any level of nested subsystems to allow the LabVIEW Simulation Interface Toolkit to map hardware to it.
      mask init:
      | NI_SIT_IO_init;
      settings: CopyFcn=NI_SIT_IO_callbacks(1);  DeleteFcn=NI_SIT_IO_callbacks(2);
      mask StyleString: edit,edit,edit,popup(auto|double|single|int8|uint8|int16|uint16|int32|uint32|boolean),popup(auto|real|complex),edit
      mask CallbackString: NI_SIT_IO_callbacks(3);|||NI_SIT_IO_callbacks(4);||
      mask TabNameString: Parameters,Parameters,Parameters,Parameters,Parameters,Parameters
      mask Display:
      | patch([-x x], [-y y], [.90980 .81960 .32156]);
      | plot([0 -x x 0], [rad -y y rad]);
      | fprintf('SIT%d', portnum);
  SIT PWM5 Servo2 : S-Function  Priority=2  FunctionName=NI_SIT_IO  Parameters=width dtype portnum stime stype btype  EnableBusSupport=off  mask(SIT Outport){portnum=2, width=-1, stime=-1, dtype=auto, stype=auto, btype=0}
      mask prompts: portnum "Port number:"; width "Port dimensions (-1 for dynamically sized):"; stime "Sample time (-1 for inherited):"; dtype "Data type:"; stype "Signal type:"; btype "Block type:"
      mask help: Use this outport on any level of nested subsystems to allow the LabVIEW Simulation Interface Toolkit to map hardware to it.
      mask init:
      | NI_SIT_IO_init;
      settings: CopyFcn=NI_SIT_IO_callbacks(1);  DeleteFcn=NI_SIT_IO_callbacks(2);
      mask StyleString: edit,edit,edit,popup(auto|double|single|int8|uint8|int16|uint16|int32|uint32|boolean),popup(auto|real|complex),edit
      mask CallbackString: NI_SIT_IO_callbacks(3);|||NI_SIT_IO_callbacks(4);||
      mask TabNameString: Parameters,Parameters,Parameters,Parameters,Parameters,Parameters
      mask Display:
      | patch([-x x], [-y y], [.90980 .81960 .32156]);
      | plot([0 -x x 0], [rad -y y rad]);
      | fprintf('SIT%d', portnum);
  SIT PWM6 Servo3 : S-Function  Priority=3  FunctionName=NI_SIT_IO  Parameters=width dtype portnum stime stype btype  EnableBusSupport=off  mask(SIT Outport){portnum=3, width=-1, stime=-1, dtype=auto, stype=auto, btype=0}
      mask prompts: portnum "Port number:"; width "Port dimensions (-1 for dynamically sized):"; stime "Sample time (-1 for inherited):"; dtype "Data type:"; stype "Signal type:"; btype "Block type:"
      mask help: Use this outport on any level of nested subsystems to allow the LabVIEW Simulation Interface Toolkit to map hardware to it.
      mask init:
      | NI_SIT_IO_init;
      settings: CopyFcn=NI_SIT_IO_callbacks(1);  DeleteFcn=NI_SIT_IO_callbacks(2);
      mask StyleString: edit,edit,edit,popup(auto|double|single|int8|uint8|int16|uint16|int32|uint32|boolean),popup(auto|real|complex),edit
      mask CallbackString: NI_SIT_IO_callbacks(3);|||NI_SIT_IO_callbacks(4);||
      mask TabNameString: Parameters,Parameters,Parameters,Parameters,Parameters,Parameters
      mask Display:
      | patch([-x x], [-y y], [.90980 .81960 .32156]);
      | plot([0 -x x 0], [rad -y y rad]);
      | fprintf('SIT%d', portnum);
  SIT PWM7 Servo4 : S-Function  Priority=4  FunctionName=NI_SIT_IO  Parameters=width dtype portnum stime stype btype  EnableBusSupport=off  mask(SIT Outport){portnum=4, width=-1, stime=-1, dtype=auto, stype=auto, btype=0}
      mask prompts: portnum "Port number:"; width "Port dimensions (-1 for dynamically sized):"; stime "Sample time (-1 for inherited):"; dtype "Data type:"; stype "Signal type:"; btype "Block type:"
      mask help: Use this outport on any level of nested subsystems to allow the LabVIEW Simulation Interface Toolkit to map hardware to it.
      mask init:
      | NI_SIT_IO_init;
      settings: CopyFcn=NI_SIT_IO_callbacks(1);  DeleteFcn=NI_SIT_IO_callbacks(2);
      mask StyleString: edit,edit,edit,popup(auto|double|single|int8|uint8|int16|uint16|int32|uint32|boolean),popup(auto|real|complex),edit
      mask CallbackString: NI_SIT_IO_callbacks(3);|||NI_SIT_IO_callbacks(4);||
      mask TabNameString: Parameters,Parameters,Parameters,Parameters,Parameters,Parameters
      mask Display:
      | patch([-x x], [-y y], [.90980 .81960 .32156]);
      | plot([0 -x x 0], [rad -y y rad]);
      | fprintf('SIT%d', portnum);
  Servo1 : Lookup2D  RowIndex=[-1,0,1]  ColumnIndex=[-1,0,1]  Table=reshape([0.06,0.0495363,0.043301,0.06,0.052446,0.043301,0.06,0.0541518,0.043301],3,3)
  Servo2 : Lookup2D  RowIndex=[-1,0,1]  ColumnIndex=[-1,0,1]  Table=reshape([0.03860880,0.0386088,0.03860880,0.0459941,0.0477243,0.0500953,0.057,0.057,0.057],3,3)
  Servo3 : Lookup2D  RowIndex=[-1,0,1]  ColumnIndex=[-1,0,1]  Table=reshape([0.0640809,0.0640809,0.0640809,0.0539629,0.0541315,0.0556492,0.0442664,0.0442664,0.0442664],3,3)
  Servo4 : Lookup2D  RowIndex=[-1,0,1]  ColumnIndex=[-1,0,1]  Table=reshape([0.0602867,0.0470489,0.0403879,0.0602867,0.049747,0.0403879,0.0602867,0.0526138,0.0403879],3,3)
  Sign : Signum
  Sum : Sum  Inputs=|++
  VPS_Power_Offset : Constant  Value=0.05
  VPS_Speed_Gain : Gain  Gain=-0.02
  VSPS Port : Gain  ParameterDataType=fixdt(1, 16)  ParameterScaling=2^0  OutDataType=fixdt(1, 16)  OutScaling=2^0
  VSPS Starboard : Gain  ParameterDataType=fixdt(1, 16)  ParameterScaling=2^0  OutDataType=fixdt(1, 16)  OutScaling=2^0
  wires:
  Sign/1 -> Product1/2, Product2/2, Product3/2, Product4/2
  Product1/1 -> -x/1  "Port VPS_X"
  Product2/1 -> -y/1  "Port VSP_Y"
  Servo1/1 -> SIT PWM4 Servo1/1
  Servo2/1 -> SIT PWM5 Servo2/1
  Product3/1 -> Servo3/1, Servo4/1  "Starboard VSP_X"
  Product4/1 -> Servo3/2, Servo4/2  "Starboard VSP_Y"
  Servo3/1 -> SIT PWM6 Servo3/1
  Servo4/1 -> SIT PWM7 Servo4/1
  VSP Speed/1 -> VPS_Speed_Gain/1, Sign/1
  VPS_Speed_Gain/1 -> Sum/1
  VPS_Power_Offset/1 -> Sum/2
  Sum/1 -> VSPS Port/1, VSPS Starboard/1
  -y/1 -> Servo2/2, Servo1/2  "Port VSP_Y"
  -x/1 -> Servo1/1, Servo2/1  "Port VPS_X"
  Starboard VSP y u_3/1 -> Product4/1
  Starboard VSP x u_4/1 -> Product3/1
  Port VSP y u_1/1 -> Product2/1
  Port VSP x u_2/1 -> Product1/1
  VSPS Port/1 -> SIT PWM1 VSPS Port/1
  VSPS Starboard/1 -> SIT PWM2 VSPS Starboard/1

== system LgV2/Plants/Linear Simulator/Linear Vessel Dynamics ==
  note: This subsystem is a modifired version of Christoffer Throvaldsens Vessel Dynamic
  tau : Inport
  D_L : Subsystem
  Initial eta : Subsystem
  Initial nu : Subsystem
  Integrator : Integrator  ExternalReset=level  InitialConditionSource=external  InitialCondition=v1_0_real  UpperSaturationLimit=velocitySatValues1  LowerSaturationLimit=-1*velocitySatValues1
  Integrator1 : Integrator  ExternalReset=level  InitialConditionSource=external  InitialCondition=eta1_0_real
  M_inv : Subsystem
  Product1 : Product  Multiplication=Matrix(*)  RndMeth=Zero
  Product2 : Product  Multiplication=Matrix(*)  RndMeth=Zero
  Product3 : Product  Multiplication=Matrix(*)  RndMeth=Zero
  R(psi) : Subsystem
  Reset Linear Simulator integrator : Constant  Value=0
  Sum : Sum  Inputs=+-
  nudot : Terminator
  psi : Selector  InputPortWidth=3  IndexOptions=Index vector (dialog)  Indices=[3]  OutputSizes=1
  eta : Outport
  nu : Outport  Port=2
  etadot : Outport  Port=3
  wires:
  Sum/1 -> Product2/2
  Product2/1 -> Integrator/1, nudot/1
  Integrator/1 -> Product1/2, nu/1, Product3/2
  R(psi)/1(R) -> Product3/1
  psi/1 -> R(psi)/1(psi)
  M_inv/1(M_inv) -> Product2/1
  tau/1 -> Sum/1
  Product1/1 -> Sum/2
  Product3/1 -> etadot/1, Integrator1/1
  Integrator1/1 -> psi/1, eta/1
  Initial nu/1(nu_0) -> Integrator/3
  Reset Linear Simulator integrator/1 -> Integrator/2, Integrator1/2
  Initial eta/1(eta_0) -> Integrator1/3
  D_L/1(D_L) -> Product1/1

== system LgV2/Control Systems/DP control/Thruster allocation/f_act to u_act ==
  f_act : Inport
  Demux : Demux  Outputs=5
  Mux : Mux  Inputs=5
  f_1 to u_1 : Subsystem
  f_2 to u_2 : Subsystem
  f_3 to u_3 : Subsystem
  f_4 to u_4 : Subsystem
  f_5 to u_5 : Subsystem
  u_act : Outport
  wires:
  f_5 to u_5/1(u_5) -> Mux/5
  f_4 to u_4/1(u_4) -> Mux/4
  f_3 to u_3/1(u_3) -> Mux/3
  f_2 to u_2/1(u_2) -> Mux/2
  f_1 to u_1/1(u_1) -> Mux/1
  Demux/5 -> f_5 to u_5/1(f_5)
  Demux/4 -> f_4 to u_4/1(f_4)
  Demux/3 -> f_3 to u_3/1(f_3)
  Demux/1 -> f_1 to u_1/1(f_1)
  Mux/1 -> u_act/1
  f_act/1 -> Demux/1
  Demux/2 -> f_2 to u_2/1(f_2)

== system LgV2/Control Systems/DP control/Thruster allocation/tau to f_act ==
  tau : Inport
  Product : Product  Multiplication=Matrix(*)  OutDataType=fixdt(1, 16)  OutScaling=2^0  RndMeth=Zero
  Pseudoinverse : dspinverses/Pseudoinverse  wanterr=off
  T_e : Subsystem
  f_act : Outport
  wires:
  Product/1 -> f_act/1
  tau/1 -> Product/2
  Pseudoinverse/1 -> Product/1
  T_e/1(T_e) -> Pseudoinverse/1

== system LgV2/Control Systems/LgV design 2/Auxilary functions g_q/g_q eq ==
  f_q : Inport
  psi_los^q : Inport  Port=2
  Product : Product  Multiplication=Matrix(*)  OutDataType=fixdt(1, 16)  OutScaling=2^0  RndMeth=Zero
  Vector Concatenate : Concatenate  Mode=Vector
  g_q : Outport
  wires:
  Vector Concatenate/1 -> g_q/1
  f_q/1 -> Vector Concatenate/1, Product/2
  psi_los^q/1 -> Product/1
  Product/1 -> Vector Concatenate/2

== system LgV2/Control Systems/LgV design 2/Auxilary functions g_q/g_q^q eq ==
  f_q : Inport
  psi_los^q : Inport  Port=2
  f_q^q : Inport  Port=3
  psi_los^q^2 : Inport  Port=4
  Add : Sum  OutDataType=fixdt(1, 16)  OutScaling=2^-10
  Matrix Concatenate : Concatenate  Mode=Multidimensional array
  Product : Product  Multiplication=Matrix(*)  OutDataType=fixdt(1, 16)  OutScaling=2^0  RndMeth=Zero
  Product1 : Product  Multiplication=Matrix(*)  OutDataType=fixdt(1, 16)  OutScaling=2^0  RndMeth=Zero
  f_q^T : dspmtrx3/Transpose  SystemSampleTime=-1  Hermitian=off  overflowFlag=off
  psi_los^q^2T : dspmtrx3/Transpose  SystemSampleTime=-1  Hermitian=off  overflowFlag=off
  g_q^q : Outport
  wires:
  f_q^q/1 -> Matrix Concatenate/1, Product1/2
  Matrix Concatenate/1 -> g_q^q/1
  Add/1 -> Matrix Concatenate/2
  f_q/1 -> f_q^T/1
  f_q^T/1 -> Product/1
  psi_los^q^2/1 -> psi_los^q^2T/1
  Product/1 -> Add/1
  psi_los^q/1 -> Product1/1
  Product1/1 -> Add/2
  psi_los^q^2T/1 -> Product/2

== system LgV2/Control Systems/LgV design 2/Auxilary functions g_q/g_q^s eq ==
  f_q : Inport
  psi_los^q : Inport  Port=2
  f_q^s : Inport  Port=3
  psi_los^qs : Inport  Port=4
  Add : Sum  OutDataType=fixdt(1, 16)  OutScaling=2^-10
  Product : Product  Multiplication=Matrix(*)  OutDataType=fixdt(1, 16)  OutScaling=2^0  RndMeth=Zero
  Product1 : Product  Multiplication=Matrix(*)  OutDataType=fixdt(1, 16)  OutScaling=2^0  RndMeth=Zero
  Vector Concatenate : Concatenate  Mode=Vector
  g_q^s : Outport
  wires:
  f_q^s/1 -> Vector Concatenate/1, Product1/2
  Vector Concatenate/1 -> g_q^s/1
  Add/1 -> Vector Concatenate/2
  Product/1 -> Add/1
  psi_los^q/1 -> Product1/1
  Product1/1 -> Add/2
  psi_los^qs/1 -> Product/1
  f_q/1 -> Product/2

== system LgV2/Control Systems/LgV design 2/Auxilary functions g_q/g_q^t eq ==
  psi_los^q : Inport
  f_q^t : Inport  Port=2
  Product1 : Product  Multiplication=Matrix(*)  OutDataType=fixdt(1, 16)  OutScaling=2^0  RndMeth=Zero
  Vector Concatenate : Concatenate  Mode=Vector
  g_q^t : Outport
  wires:
  f_q^t/1 -> Vector Concatenate/1, Product1/2
  Vector Concatenate/1 -> g_q^t/1
  Product1/1 -> Vector Concatenate/2
  psi_los^q/1 -> Product1/1

== system LgV2/Control Systems/LgV design 2/Auxiliary function g_s/g_s eq ==
  f_s : Inport
  psi_los^s : Inport  Port=2
  0_2x1 : Constant  Value=[0;0]  VectorParams1D=off  OutDataType=fixdt(1, 16)  OutScaling=2^0
  Product : Product  Multiplication=Matrix(*)  OutDataType=fixdt(1, 16)  OutScaling=2^0  RndMeth=Zero
  Vector Concatenate : Concatenate  Mode=Vector
  g_s : Outport
  wires:
  Vector Concatenate/1 -> g_s/1
  f_s/1 -> Product/2
  psi_los^s/1 -> Product/1
  Product/1 -> Vector Concatenate/2
  0_2x1/1 -> Vector Concatenate/1

== system LgV2/Control Systems/LgV design 2/Auxiliary function g_s/g_s^q eq ==
  f_s : Inport
  psi_los^s : Inport  Port=2
  f_s^q : Inport  Port=3
  psi_los^sq : Inport  Port=4
  0_2x2 : Constant  Value=[0 0; 0 0]  VectorParams1D=off  OutDataType=fixdt(1, 16)  OutScaling=2^0
  Add : Sum  OutDataType=fixdt(1, 16)  OutScaling=2^-10
  Matrix Concatenate : Concatenate  Mode=Multidimensional array
  Product : Product  OutDataType=fixdt(1, 16)  OutScaling=2^0  RndMeth=Zero
  Product1 : Product  OutDataType=fixdt(1, 16)  OutScaling=2^0  RndMeth=Zero
  g_s^q : Outport
  wires:
  Matrix Concatenate/1 -> g_s^q/1
  Add/1 -> Matrix Concatenate/2
  Product/1 -> Add/1
  psi_los^s/1 -> Product1/1
  Product1/1 -> Add/2
  0_2x2/1 -> Matrix Concatenate/1
  f_s^q/1 -> Product1/2
  psi_los^sq/1 -> Product/1
  f_s/1 -> Product/2

== system LgV2/Control Systems/LgV design 2/Auxiliary function g_s/g_s^s eq ==
  f_s : Inport
  psi_los^s : Inport  Port=2
  f_s^s : Inport  Port=3
  psi_los^s^2 : Inport  Port=4
  0_2x1 : Constant  Value=[0;0]  VectorParams1D=off  OutDataType=fixdt(1, 16)  OutScaling=2^0
  Add : Sum  OutDataType=fixdt(1, 16)  OutScaling=2^-10
  Product : Product  OutDataType=fixdt(1, 16)  OutScaling=2^0  RndMeth=Zero
  Product1 : Product  OutDataType=fixdt(1, 16)  OutScaling=2^0  RndMeth=Zero
  Vector Concatenate : Concatenate  Mode=Vector
  g_s^s : Outport
  wires:
  Vector Concatenate/1 -> g_s^s/1
  Add/1 -> Vector Concatenate/2
  Product/1 -> Add/1
  psi_los^s/1 -> Product1/1
  Product1/1 -> Add/2
  psi_los^s^2/1 -> Product/1
  f_s/1 -> Product/2
  0_2x1/1 -> Vector Concatenate/1
  f_s^s/1 -> Product1/2

== system LgV2/Control Systems/LgV design 2/Auxiliary function g_s/g_s^t eq ==
  psi_los^s : Inport
  f_s^t : Inport  Port=2
  0_2x1 : Constant  Value=[0;0]  VectorParams1D=off  OutDataType=fixdt(1, 16)  OutScaling=2^0
  Product1 : Product  Multiplication=Matrix(*)  OutDataType=fixdt(1, 16)  OutScaling=2^0  RndMeth=Zero
  Vector Concatenate : Concatenate  Mode=Vector
  g_a^t : Outport
  wires:
  Vector Concatenate/1 -> g_a^t/1
  Product1/1 -> Vector Concatenate/2
  psi_los^s/1 -> Product1/1
  0_2x1/1 -> Vector Concatenate/1
  f_s^t/1 -> Product1/2

== system LgV2/Control Systems/LgV design 2/Control law/D_L ==
  -N_r : Gain  Gain=-1  ParameterDataType=fixdt(1, 16)  ParameterScaling=2^0  OutDataType=fixdt(1, 16)  OutScaling=2^0
  -N_v : Gain  Gain=-1  ParameterDataType=fixdt(1, 16)  ParameterScaling=2^0  OutDataType=fixdt(1, 16)  OutScaling=2^0
  -X_u : Gain  Gain=-1  ParameterDataType=fixdt(1, 16)  ParameterScaling=2^0  OutDataType=fixdt(1, 16)  OutScaling=2^0
  -Y_v : Gain  Gain=-1  ParameterDataType=fixdt(1, 16)  ParameterScaling=2^0  OutDataType=fixdt(1, 16)  OutScaling=2^0
  -Y_vr : Gain  Gain=-1  ParameterDataType=fixdt(1, 16)  ParameterScaling=2^0  OutDataType=fixdt(1, 16)  OutScaling=2^0
  D_L_{12..13,21,31} (4 alike) : Constant  Value=0
  Linear Dampning matrix : Reshape  OutputDimensionality=Customize  OutputDimensions=[3,3]
  Mux : Mux  Inputs=9
  N_r : Constant  Value=-1.900
  N_v : Constant  Value=0.18140
  X_u : Constant  Value=-0.59739
  Y_r : Constant  Value=-7.250
  Y_v : Constant  Value=-3.50625
  D_L : Outport
  wires:
  -N_r/1 -> Mux/9
  -Y_vr/1 -> Mux/8
  D_L_13/1 -> Mux/7
  -N_v/1 -> Mux/6
  -Y_v/1 -> Mux/5
  D_L_12/1 -> Mux/4
  D_L_31/1 -> Mux/3
  D_L_21/1 -> Mux/2
  -X_u/1 -> Mux/1
  N_r/1 -> -N_r/1
  Y_r/1 -> -Y_vr/1
  N_v/1 -> -N_v/1
  Y_v/1 -> -Y_v/1
  Linear Dampning matrix/1 -> D_L/1
  Mux/1 -> Linear Dampning matrix/1
  X_u/1 -> -X_u/1

== system LgV2/Control Systems/LgV design 2/Thruster allocation/f_act to u_act ==
  f_act : Inport
  Demux : Demux  Outputs=5
  Mux : Mux  Inputs=5
  f_1 to u_1 : Subsystem
  f_2 to u_2 : Subsystem
  f_3 to u_3 : Subsystem
  f_4 to u_4 : Subsystem
  f_5 to u_5 : Subsystem
  u_act : Outport
  wires:
  f_5 to u_5/1(u_5) -> Mux/5
  f_4 to u_4/1(u_4) -> Mux/4
  f_3 to u_3/1(u_3) -> Mux/3
  f_2 to u_2/1(u_2) -> Mux/2
  f_1 to u_1/1(u_1) -> Mux/1
  Demux/5 -> f_5 to u_5/1(f_5)
  Demux/4 -> f_4 to u_4/1(f_4)
  Demux/3 -> f_3 to u_3/1(f_3)
  Demux/1 -> f_1 to u_1/1(f_1)
  Mux/1 -> u_act/1
  f_act/1 -> Demux/1
  Demux/2 -> f_2 to u_2/1(f_2)

== system LgV2/Control Systems/LgV design 2/Thruster allocation/tau to f_act ==
  tau : Inport
  Product : Product  Multiplication=Matrix(*)  OutDataType=fixdt(1, 16)  OutScaling=2^0  RndMeth=Zero
  Pseudoinverse : dspinverses/Pseudoinverse  wanterr=off
  T_e : Subsystem
  f_act : Outport
  wires:
  Product/1 -> f_act/1
  tau/1 -> Product/2
  Pseudoinverse/1 -> Product/1
  T_e/1(T_e) -> Pseudoinverse/1

== system LgV2/Control Systems/LgV design 2/Update laws/q_0 ==
  Mux : Mux  Inputs=2
  q_x_0 : Constant  Value=0  OutDataType=fixdt(1, 16)  OutScaling=2^0
  q_y_0 : Constant  Value=0  OutDataType=fixdt(1, 16)  OutScaling=2^0
  q_0 : Outport  OutDataType=fixdt(1, 16)  OutScaling=2^0
  wires:
  q_x_0/1 -> Mux/1
  q_y_0/1 -> Mux/2
  Mux/1 -> q_0/1

== system LgV2/Control Systems/LgV design 2/z_1 eq/heading to pipi ==
  In1 : Inport
  Demux : Demux  Outputs=3
  Mux : Mux  Inputs=3
  rad to pi2pi : Subsystem  AncestorBlock=marine_gnc/Utilities/Math Operations/deg to 180//180
      mask Type: rad to pi/pi
      mask Description: Converts an angle in rad to +- pi
      mask Display: disp('[0 2pi] to [-pi pi]')
  Out1 : Outport
  wires:
  Demux/3 -> rad to pi2pi/1(x (rad))
  Demux/1 -> Mux/1
  Demux/2 -> Mux/2
  rad to pi2pi/1(-pi to pi) -> Mux/3
  In1/1 -> Demux/1
  Mux/1 -> Out1/1

== system LgV2/Control Systems/LgV design 2/z_1 eq/heading to pipi1 ==
  In1 : Inport
  Demux : Demux  Outputs=3
  Mux : Mux  Inputs=3
  Scope : Scope
      settings: SaveName=ScopeData6
  rad to pi2pi : Subsystem  AncestorBlock=marine_gnc/Utilities/Math Operations/deg to 180//180
      mask Type: rad to pi/pi
      mask Description: Converts an angle in rad to +- pi
      mask Display: disp('[0 2pi] to [-pi pi]')
  Out1 : Outport
  wires:
  Demux/3 -> rad to pi2pi/1(x (rad))
  Demux/1 -> Mux/1
  Demux/2 -> Mux/2
  rad to pi2pi/1(-pi to pi) -> Mux/3, Scope/1
  In1/1 -> Demux/1
  Mux/1 -> Out1/1
